simulink model "CLLC_simu"  (R2025b)
settings: Solver=ode23tb  StartTime=0.0  StopTime=simlength  MaxStep=tc  RelTol=1e-3
values from neighbouring files (symbols this model uses):
  alpha1 = 0    [init.m]    (also in state_space_equations.m = linspace(pi/2,pi,3))
  alpha2 = 0    [init.m]    (also in state_space_equations.m = linspace(pi/2,pi,3))
  fr = 1/(2*pi*sqrt(Lr1*Cr1))    [init.m]
  phase_shift = pi/6    (= 0.523598775598)    [init.m]
  R1 = 0.026    [Optimal_Design_CLLLC.m]    (also in init.m = 0.1; state_space_equations.m = 0.1)
  R2 = 0.026    [Optimal_Design_CLLLC.m]    (also in init.m = 0.1; state_space_equations.m = 0.1)
  Td = 0.015 * Ts    (= 1.66666666667e-07)    [init.m]
libraries: fl_lib x60, nesl_utility x35, ee_lib x2, eeGeneralControl x1, single_phase_transformer x1
(part 2 of 2)

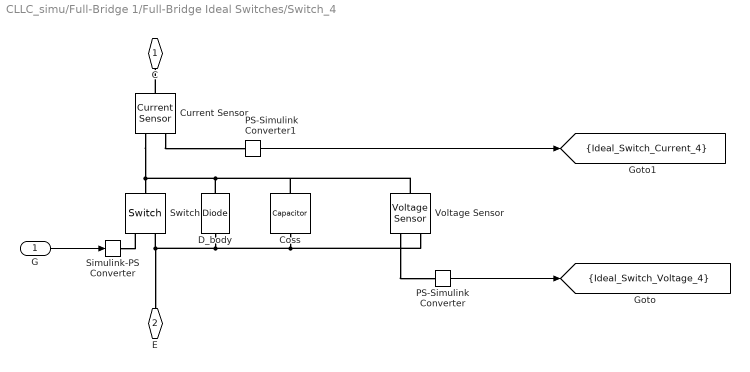
== system CLLC_simu/Full-Bridge 1/Full-Bridge Ideal Switches/Switch_4 ==
  G : Inport
  Coss : fl_lib/Electrical/Electrical Elements/Capacitor  c=1e-9 F  r=1e-6 Ohm  g=0 1/Ohm  i_specify=off  i_priority=None  i=0 A  i_nominal_specify=off  i_nominal_value=1  i_nominal_unit=A  v_specify=off  v_priority=None  v=0 V  v_nominal_specify=off  v_nominal_value=1  v_nominal_unit=V  vc_specify=off  vc_priority=High  vc=0 V  vc_nominal_specify=off  vc_nominal_value=1  vc_nominal_unit=V
  Current Sensor : fl_lib/Electrical/Electrical Sensors/Current Sensor
  D_body : fl_lib/Electrical/Electrical Elements/Diode  Vf=0.6 V  Ron=15e-4 Ohm  Goff=1e-8 1/Ohm  i_specify=off  i_priority=None  i=0 A  i_nominal_specify=off  i_nominal_value=1  i_nominal_unit=A  v_specify=off  v_priority=None  v=0 V  v_nominal_specify=off  v_nominal_value=1  v_nominal_unit=V
  PS-Simulink Converter : nesl_utility/PS-Simulink Converter  PhysicalDomain=network_engine_domain  SubClassName=ps_output  LeftPortType=input  RightPortType=output  PseudoPeriodic=off  Frequencies=[]  VectorFormat=inherit  Unit=inherit  AffineConversion=off
  PS-Simulink Converter1 : nesl_utility/PS-Simulink Converter  PhysicalDomain=network_engine_domain  SubClassName=ps_output  LeftPortType=input  RightPortType=output  PseudoPeriodic=off  Frequencies=[]  VectorFormat=inherit  Unit=inherit  AffineConversion=off
  Simulink-PS Converter : nesl_utility/Simulink-PS Converter  PhysicalDomain=network_engine_domain  SubClassName=ps_input  LeftPortType=input  RightPortType=output  PseudoPeriodic=off  Frequencies=[]  NoiseDistribution=none  NoiseParameters=[]  Unit=1  AffineConversion=off  FilteringAndDerivatives=provide  SimscapeFilterOrder=1  InputFilterTimeConstant=0.001  UdotUserProvided=0
  Switch : fl_lib/Electrical/Electrical Elements/Switch  R_closed=0.01 Ohm  G_open=1e-8 1/Ohm  Threshold=0.5  i_specify=off  i_priority=None  i=0 A  i_nominal_specify=off  i_nominal_value=1  i_nominal_unit=A  v_specify=off  v_priority=None  v=0 V  v_nominal_specify=off  v_nominal_value=1  v_nominal_unit=V
  Voltage Sensor : fl_lib/Electrical/Electrical Sensors/Voltage Sensor
  C : PMIOPort  Side=Left
  E : PMIOPort  Port=2  Side=Right
  tag scope: Ideal_Switch_Current_4=scoped, Ideal_Switch_Voltage_4=scoped
  wires:
  PS-Simulink Converter1/1 -> [Ideal_Switch_Current_4]
  PS-Simulink Converter/1 -> [Ideal_Switch_Voltage_4]
  G/1 -> Simulink-PS Converter/1
  connections:
  Current Sensor/RConn1 -- PS-Simulink Converter1/LConn1
  Current Sensor/LConn1 -- C/RConn1
  Voltage Sensor/RConn1 -- PS-Simulink Converter/LConn1
  Simulink-PS Converter/RConn1 -- Switch/RConn1
  Current Sensor/RConn2 -- Switch/LConn1 -- D_body/RConn1 -- Coss/LConn1 -- Voltage Sensor/LConn1
  Coss/RConn1 -- Voltage Sensor/RConn2 -- D_body/LConn1 -- Switch/RConn2 -- E/RConn1

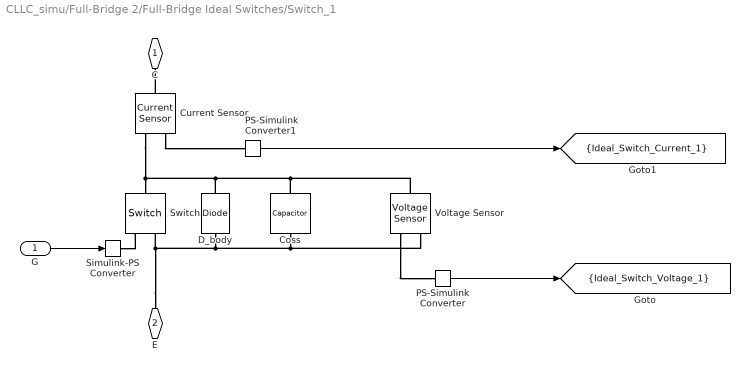
== system CLLC_simu/Full-Bridge 2/Full-Bridge Ideal Switches/Switch_1 ==
  G : Inport
  Coss : fl_lib/Electrical/Electrical Elements/Capacitor  c=1e-9 F  r=1e-6 Ohm  g=0 1/Ohm  i_specify=off  i_priority=None  i=0 A  i_nominal_specify=off  i_nominal_value=1  i_nominal_unit=A  v_specify=off  v_priority=None  v=0 V  v_nominal_specify=off  v_nominal_value=1  v_nominal_unit=V  vc_specify=off  vc_priority=High  vc=0 V  vc_nominal_specify=off  vc_nominal_value=1  vc_nominal_unit=V
  Current Sensor : fl_lib/Electrical/Electrical Sensors/Current Sensor
  D_body : fl_lib/Electrical/Electrical Elements/Diode  Vf=0.6 V  Ron=15e-4 Ohm  Goff=1e-8 1/Ohm  i_specify=off  i_priority=None  i=0 A  i_nominal_specify=off  i_nominal_value=1  i_nominal_unit=A  v_specify=off  v_priority=None  v=0 V  v_nominal_specify=off  v_nominal_value=1  v_nominal_unit=V
  PS-Simulink Converter : nesl_utility/PS-Simulink Converter  PhysicalDomain=network_engine_domain  SubClassName=ps_output  LeftPortType=input  RightPortType=output  PseudoPeriodic=off  Frequencies=[]  VectorFormat=inherit  Unit=inherit  AffineConversion=off
  PS-Simulink Converter1 : nesl_utility/PS-Simulink Converter  PhysicalDomain=network_engine_domain  SubClassName=ps_output  LeftPortType=input  RightPortType=output  PseudoPeriodic=off  Frequencies=[]  VectorFormat=inherit  Unit=inherit  AffineConversion=off
  Simulink-PS Converter : nesl_utility/Simulink-PS Converter  PhysicalDomain=network_engine_domain  SubClassName=ps_input  LeftPortType=input  RightPortType=output  PseudoPeriodic=off  Frequencies=[]  NoiseDistribution=none  NoiseParameters=[]  Unit=1  AffineConversion=off  FilteringAndDerivatives=provide  SimscapeFilterOrder=1  InputFilterTimeConstant=0.001  UdotUserProvided=0
  Switch : fl_lib/Electrical/Electrical Elements/Switch  R_closed=0.01 Ohm  G_open=1e-8 1/Ohm  Threshold=0.5  i_specify=off  i_priority=None  i=0 A  i_nominal_specify=off  i_nominal_value=1  i_nominal_unit=A  v_specify=off  v_priority=None  v=0 V  v_nominal_specify=off  v_nominal_value=1  v_nominal_unit=V
  Voltage Sensor : fl_lib/Electrical/Electrical Sensors/Voltage Sensor
  C : PMIOPort  Side=Left
  E : PMIOPort  Port=2  Side=Right
  tag scope: Ideal_Switch_Current_1=scoped, Ideal_Switch_Voltage_1=scoped
  wires:
  G/1 -> Simulink-PS Converter/1
  PS-Simulink Converter/1 -> [Ideal_Switch_Voltage_1]
  PS-Simulink Converter1/1 -> [Ideal_Switch_Current_1]
  connections:
  E/RConn1 -- Switch/RConn2 -- D_body/LConn1 -- Voltage Sensor/RConn2 -- Coss/RConn1
  Voltage Sensor/LConn1 -- Coss/LConn1 -- D_body/RConn1 -- Switch/LConn1 -- Current Sensor/RConn2
  Simulink-PS Converter/RConn1 -- Switch/RConn1
  Voltage Sensor/RConn1 -- PS-Simulink Converter/LConn1
  Current Sensor/LConn1 -- C/RConn1
  Current Sensor/RConn1 -- PS-Simulink Converter1/LConn1

== system CLLC_simu/Full-Bridge 2/Full-Bridge Ideal Switches/Switch_2 ==
  G : Inport
  Coss : fl_lib/Electrical/Electrical Elements/Capacitor  c=1e-9 F  r=1e-6 Ohm  g=0 1/Ohm  i_specify=off  i_priority=None  i=0 A  i_nominal_specify=off  i_nominal_value=1  i_nominal_unit=A  v_specify=off  v_priority=None  v=0 V  v_nominal_specify=off  v_nominal_value=1  v_nominal_unit=V  vc_specify=off  vc_priority=High  vc=0 V  vc_nominal_specify=off  vc_nominal_value=1  vc_nominal_unit=V
  Current Sensor : fl_lib/Electrical/Electrical Sensors/Current Sensor
  D_body : fl_lib/Electrical/Electrical Elements/Diode  Vf=0.6 V  Ron=15e-4 Ohm  Goff=1e-8 1/Ohm  i_specify=off  i_priority=None  i=0 A  i_nominal_specify=off  i_nominal_value=1  i_nominal_unit=A  v_specify=off  v_priority=None  v=0 V  v_nominal_specify=off  v_nominal_value=1  v_nominal_unit=V
  PS-Simulink Converter : nesl_utility/PS-Simulink Converter  PhysicalDomain=network_engine_domain  SubClassName=ps_output  LeftPortType=input  RightPortType=output  PseudoPeriodic=off  Frequencies=[]  VectorFormat=inherit  Unit=inherit  AffineConversion=off
  PS-Simulink Converter1 : nesl_utility/PS-Simulink Converter  PhysicalDomain=network_engine_domain  SubClassName=ps_output  LeftPortType=input  RightPortType=output  PseudoPeriodic=off  Frequencies=[]  VectorFormat=inherit  Unit=inherit  AffineConversion=off
  Simulink-PS Converter : nesl_utility/Simulink-PS Converter  PhysicalDomain=network_engine_domain  SubClassName=ps_input  LeftPortType=input  RightPortType=output  PseudoPeriodic=off  Frequencies=[]  NoiseDistribution=none  NoiseParameters=[]  Unit=1  AffineConversion=off  FilteringAndDerivatives=provide  SimscapeFilterOrder=1  InputFilterTimeConstant=0.001  UdotUserProvided=0
  Switch : fl_lib/Electrical/Electrical Elements/Switch  R_closed=0.01 Ohm  G_open=1e-8 1/Ohm  Threshold=0.5  i_specify=off  i_priority=None  i=0 A  i_nominal_specify=off  i_nominal_value=1  i_nominal_unit=A  v_specify=off  v_priority=None  v=0 V  v_nominal_specify=off  v_nominal_value=1  v_nominal_unit=V
  Voltage Sensor : fl_lib/Electrical/Electrical Sensors/Voltage Sensor
  C : PMIOPort  Side=Left
  E : PMIOPort  Port=2  Side=Right
  tag scope: Ideal_Switch_Current_2=scoped, Ideal_Switch_Voltage_2=scoped
  wires:
  PS-Simulink Converter1/1 -> [Ideal_Switch_Current_2]
  PS-Simulink Converter/1 -> [Ideal_Switch_Voltage_2]
  G/1 -> Simulink-PS Converter/1
  connections:
  Current Sensor/RConn1 -- PS-Simulink Converter1/LConn1
  Current Sensor/LConn1 -- C/RConn1
  Voltage Sensor/RConn1 -- PS-Simulink Converter/LConn1
  Simulink-PS Converter/RConn1 -- Switch/RConn1
  Current Sensor/RConn2 -- Switch/LConn1 -- D_body/RConn1 -- Coss/LConn1 -- Voltage Sensor/LConn1
  Coss/RConn1 -- Voltage Sensor/RConn2 -- D_body/LConn1 -- Switch/RConn2 -- E/RConn1

== system CLLC_simu/Full-Bridge 2/Full-Bridge Ideal Switches/Switch_3 ==
  G : Inport
  Coss : fl_lib/Electrical/Electrical Elements/Capacitor  c=1e-9 F  r=1e-6 Ohm  g=0 1/Ohm  i_specify=off  i_priority=None  i=0 A  i_nominal_specify=off  i_nominal_value=1  i_nominal_unit=A  v_specify=off  v_priority=None  v=0 V  v_nominal_specify=off  v_nominal_value=1  v_nominal_unit=V  vc_specify=off  vc_priority=High  vc=0 V  vc_nominal_specify=off  vc_nominal_value=1  vc_nominal_unit=V
  Current Sensor : fl_lib/Electrical/Electrical Sensors/Current Sensor
  D_body : fl_lib/Electrical/Electrical Elements/Diode  Vf=0.6 V  Ron=15e-4 Ohm  Goff=1e-8 1/Ohm  i_specify=off  i_priority=None  i=0 A  i_nominal_specify=off  i_nominal_value=1  i_nominal_unit=A  v_specify=off  v_priority=None  v=0 V  v_nominal_specify=off  v_nominal_value=1  v_nominal_unit=V
  PS-Simulink Converter : nesl_utility/PS-Simulink Converter  PhysicalDomain=network_engine_domain  SubClassName=ps_output  LeftPortType=input  RightPortType=output  PseudoPeriodic=off  Frequencies=[]  VectorFormat=inherit  Unit=inherit  AffineConversion=off
  PS-Simulink Converter1 : nesl_utility/PS-Simulink Converter  PhysicalDomain=network_engine_domain  SubClassName=ps_output  LeftPortType=input  RightPortType=output  PseudoPeriodic=off  Frequencies=[]  VectorFormat=inherit  Unit=inherit  AffineConversion=off
  Simulink-PS Converter : nesl_utility/Simulink-PS Converter  PhysicalDomain=network_engine_domain  SubClassName=ps_input  LeftPortType=input  RightPortType=output  PseudoPeriodic=off  Frequencies=[]  NoiseDistribution=none  NoiseParameters=[]  Unit=1  AffineConversion=off  FilteringAndDerivatives=provide  SimscapeFilterOrder=1  InputFilterTimeConstant=0.001  UdotUserProvided=0
  Switch : fl_lib/Electrical/Electrical Elements/Switch  R_closed=0.01 Ohm  G_open=1e-8 1/Ohm  Threshold=0.5  i_specify=off  i_priority=None  i=0 A  i_nominal_specify=off  i_nominal_value=1  i_nominal_unit=A  v_specify=off  v_priority=None  v=0 V  v_nominal_specify=off  v_nominal_value=1  v_nominal_unit=V
  Voltage Sensor : fl_lib/Electrical/Electrical Sensors/Voltage Sensor
  C : PMIOPort  Side=Left
  E : PMIOPort  Port=2  Side=Right
  tag scope: Ideal_Switch_Current_3=scoped, Ideal_Switch_Voltage_3=scoped
  wires:
  G/1 -> Simulink-PS Converter/1
  PS-Simulink Converter/1 -> [Ideal_Switch_Voltage_3]
  PS-Simulink Converter1/1 -> [Ideal_Switch_Current_3]
  connections:
  E/RConn1 -- Switch/RConn2 -- D_body/LConn1 -- Voltage Sensor/RConn2 -- Coss/RConn1
  Voltage Sensor/LConn1 -- Coss/LConn1 -- D_body/RConn1 -- Switch/LConn1 -- Current Sensor/RConn2
  Simulink-PS Converter/RConn1 -- Switch/RConn1
  Voltage Sensor/RConn1 -- PS-Simulink Converter/LConn1
  Current Sensor/LConn1 -- C/RConn1
  Current Sensor/RConn1 -- PS-Simulink Converter1/LConn1

== system CLLC_simu/Full-Bridge 2/Full-Bridge Ideal Switches/Switch_4 ==
  G : Inport
  Coss : fl_lib/Electrical/Electrical Elements/Capacitor  c=1e-9 F  r=1e-6 Ohm  g=0 1/Ohm  i_specify=off  i_priority=None  i=0 A  i_nominal_specify=off  i_nominal_value=1  i_nominal_unit=A  v_specify=off  v_priority=None  v=0 V  v_nominal_specify=off  v_nominal_value=1  v_nominal_unit=V  vc_specify=off  vc_priority=High  vc=0 V  vc_nominal_specify=off  vc_nominal_value=1  vc_nominal_unit=V
  Current Sensor : fl_lib/Electrical/Electrical Sensors/Current Sensor
  D_body : fl_lib/Electrical/Electrical Elements/Diode  Vf=0.6 V  Ron=15e-4 Ohm  Goff=1e-8 1/Ohm  i_specify=off  i_priority=None  i=0 A  i_nominal_specify=off  i_nominal_value=1  i_nominal_unit=A  v_specify=off  v_priority=None  v=0 V  v_nominal_specify=off  v_nominal_value=1  v_nominal_unit=V
  PS-Simulink Converter : nesl_utility/PS-Simulink Converter  PhysicalDomain=network_engine_domain  SubClassName=ps_output  LeftPortType=input  RightPortType=output  PseudoPeriodic=off  Frequencies=[]  VectorFormat=inherit  Unit=inherit  AffineConversion=off
  PS-Simulink Converter1 : nesl_utility/PS-Simulink Converter  PhysicalDomain=network_engine_domain  SubClassName=ps_output  LeftPortType=input  RightPortType=output  PseudoPeriodic=off  Frequencies=[]  VectorFormat=inherit  Unit=inherit  AffineConversion=off
  Simulink-PS Converter : nesl_utility/Simulink-PS Converter  PhysicalDomain=network_engine_domain  SubClassName=ps_input  LeftPortType=input  RightPortType=output  PseudoPeriodic=off  Frequencies=[]  NoiseDistribution=none  NoiseParameters=[]  Unit=1  AffineConversion=off  FilteringAndDerivatives=provide  SimscapeFilterOrder=1  InputFilterTimeConstant=0.001  UdotUserProvided=0
  Switch : fl_lib/Electrical/Electrical Elements/Switch  R_closed=0.01 Ohm  G_open=1e-8 1/Ohm  Threshold=0.5  i_specify=off  i_priority=None  i=0 A  i_nominal_specify=off  i_nominal_value=1  i_nominal_unit=A  v_specify=off  v_priority=None  v=0 V  v_nominal_specify=off  v_nominal_value=1  v_nominal_unit=V
  Voltage Sensor : fl_lib/Electrical/Electrical Sensors/Voltage Sensor
  C : PMIOPort  Side=Left
  E : PMIOPort  Port=2  Side=Right
  tag scope: Ideal_Switch_Current_4=scoped, Ideal_Switch_Voltage_4=scoped
  wires:
  PS-Simulink Converter1/1 -> [Ideal_Switch_Current_4]
  PS-Simulink Converter/1 -> [Ideal_Switch_Voltage_4]
  G/1 -> Simulink-PS Converter/1
  connections:
  Current Sensor/RConn1 -- PS-Simulink Converter1/LConn1
  Current Sensor/LConn1 -- C/RConn1
  Voltage Sensor/RConn1 -- PS-Simulink Converter/LConn1
  Simulink-PS Converter/RConn1 -- Switch/RConn1
  Current Sensor/RConn2 -- Switch/LConn1 -- D_body/RConn1 -- Coss/LConn1 -- Voltage Sensor/LConn1
  Coss/RConn1 -- Voltage Sensor/RConn2 -- D_body/LConn1 -- Switch/RConn2 -- E/RConn1

== matlab function CLLC_simu/Controller/PWM Generator/MATLAB Function ==
  data: phase input; y output; frequency input; time input
function y = fcn(phase,frequency,time)
time_offset = (phase / 2/pi) / frequency;
y = mod(time + time_offset, 1/frequency) * frequency;

== matlab function CLLC_simu/Controller/PWM Generator/MATLAB Function2 ==
  data: phase input; y output; frequency input; time input
function y = fcn(phase,frequency,time)
time_offset = (phase / 2/pi) / frequency;
y = mod(time + time_offset, 1/frequency) * frequency;

== matlab function CLLC_simu/Controller/PWM Generator/MATLAB Function3 ==
  data: phase input; y output; frequency input; time input
function y = fcn(phase,frequency,time)
time_offset = (phase / 2/pi) / frequency;
y = mod(time + time_offset, 1/frequency) * frequency;

== matlab function CLLC_simu/Controller/PWM Generator/MATLAB Function4 ==
  data: phase input; y output; frequency input; time input
function y = fcn(phase,frequency,time)
time_offset = (phase / 2/pi) / frequency;
y = mod(time + time_offset, 1/frequency) * frequency;

== matlab function CLLC_simu/Controller/PWM Generator/MATLAB Function5 ==
  data: phase input; y output; frequency input; time input
function y = fcn(phase,frequency,time)
time_offset = (phase / 2/pi) / frequency;
y = mod(time + time_offset, 1/frequency) * frequency;

== matlab function CLLC_simu/Controller/PWM Generator/MATLAB Function6 ==
  data: phase input; y output; frequency input; time input
function y = fcn(phase,frequency,time)
time_offset = (phase / 2/pi) / frequency;
y = mod(time + time_offset, 1/frequency) * frequency;

== matlab function CLLC_simu/Controller/PWM Generator/MATLAB Function7 ==
  data: phase input; y output; frequency input; time input
function y = fcn(phase,frequency,time)
time_offset = (phase / 2/pi) / frequency;
y = mod(time + time_offset, 1/frequency) * frequency;

== matlab function CLLC_simu/Controller/PWM Generator/MATLAB Function1 ==
  data: phase input; y output; frequency input; time input
function y = fcn(phase,frequency,time)
time_offset = (phase / 2/pi) / frequency;
y = mod(time + time_offset, 1/frequency) * frequency;
